simulink model "robot_model_with_torque"  (R2018b)
settings: Solver=VariableStepAuto  StartTime=0.0  StopTime=25  RelTol=1e-6
model workspace: external: MATLAB File load_data.m (data not in the file)
values from neighbouring files (symbols this model uses):
  m = [5.70044 3.22698 4.31272 2.07206 2.24665 1.60879]    [init_robot.m]    (also in load_data.m)
  smiData = struct    [load_data.m]
undefined symbols (not defined in the file or in its folder): X, Y, Z
libraries: sm_lib x40, nesl_utility x15, simulink x1
(part 2 of 2)

== matlab function robot_model_with_torque/motores1/MATLAB Function5 ==
  data: E output; Y input; dY input; iE input; U output; Yref input; dYref input; k input
function [E,U] = PID(Y,dY,iE,Yref,dYref,k)

E = Yref - Y;
dE = dYref - dY;

U = k(1)*E + k(2)*iE + k(3)*dE;

== matlab function robot_model_with_torque/motores1/MATLAB Function6 ==
  data: U input; D input; dX output; Y output; X input
function [dX,Y]= motor_modelo(U,D,X)

%MATRICES DEL MOTOR
Ra = 11.24;
La = 2.713e-3;
Kb = 14.87e-3;
Kt = Kb;
bm = 2.01e-6;
Jm = 2779.56e-9;

A = [-Ra/La -Kb/La;Kt/Jm -bm/Jm];
B = [1/La;0];
C = [0 1];

%CONTROLADOR PID
dX = [A*X + B*U];
Y = [C*X + D*U];

== matlab function robot_model_with_torque/motores1/MATLAB Function7 ==
  data: E output; Y input; dY input; iE input; U output; Yref input; dYref input; k input
function [E,U] = PID(Y,dY,iE,Yref,dYref,k)

E = Yref - Y;
dE = dYref - dY;

U = k(1)*E + k(2)*iE + k(3)*dE;

== matlab function robot_model_with_torque/motores1/MATLAB Function8 ==
  data: U input; D input; dX output; Y output; X input
function [dX,Y]= motor_modelo(U,D,X)

%MATRICES DEL MOTOR
Ra = 11.24;
La = 2.713e-3;
Kb = 14.87e-3;
Kt = Kb;
bm = 2.01e-6;
Jm = 2779.56e-9;

A = [-Ra/La -Kb/La;Kt/Jm -bm/Jm];
B = [1/La;0];
C = [0 1];

%CONTROLADOR PID
dX = [A*X + B*U];
Y = [C*X + D*U];

== matlab function robot_model_with_torque/motores1/MATLAB Function9 ==
  data: w output; q input; dq input; torque output; ddq input; dw input
function [w,torque] = fcn(q, dq, ddq, dw)

d = [0.2703 0 0.3644 0 0.3743 0 0.2295]; %metros
a = [0.069 0 0.069 0 0.01 0 0]; %matros
alpha = [-pi/2 pi/2 -pi/2 pi/2 -pi/2 pi/2 0]; %radianes
m = [5.70044 3.22698 4.31272 2.07206 2.24665 1.60879 0.54218]; %kg

xc = [-0.05117 0.00269 -0.07176 0.00159 -0.01168 0.00697 0.005137]; %metros
yc = [0.07908 -0.00529 0.08149 -0.01117 0.13111 0.006 0.0009572];
zc = [0.00086 0.06845 0.00132 0.02618 0.0046 0.06048 0.0-6682];

%Tensores de inercia (kg*m^2)
Ixx = [0.047091023 0.027885975 0.026617336 0.013182279 0.016677428 0.007005379 0.000816214];
Iyy = [0.035959884 0.020787492 0.012480083 0.00926852 0.003746311 0.005527552 0.000873501];
Izz = [0.037669765 0.011752094 0.028443552 0.007115827 0.016754573 0.003876072 0.000549415];
Ixy = [-0.0061487 -0.00018822 -0.003921899 -0.000196634 -0.000186576 0.000153481 0.00012844];
Iyx = [-0.0061487 -0.00018822 -0.003921899 -0.000196634 -0.000186576 0.000153481 0.00012844];
Iyz = [-0.000780869 0.002076758 -0.001083893 0.000745949 0.000647324 -0.00021115 0.000105773];
Izy = [-0.000780869 0.002076758 -0.001083893 0.000745949 0.000647324 -0.00021115 0.000105773];
Ixz = [0.000127876 -0.000300964 0.000292706 0.000360362 0.000184037 -0.000443848 0.000189699];
Izx = [0.000127876 -0.000300964 0.000292706 0.000360362 0.000184037 -0.000443848 0.000189699];

Ti = denavit_hartenberg(q,a,alpha,d,0,7);
rici = zeros(3,7);
rmci = zeros(3,7);
rimi = zeros(3,7);

for i = 1:7
    rici(:,i) = Ti{i}(1:3,4)- [xc(i);yc(i);zc(i)];
end

for i = 1:6
    rmci(:,i) = Ti{i + 1}(1:3,4)- Ti{i}(1:3,4) - [xc(i);yc(i);zc(i)];
end

for i = 1:6
    rimi(:,i) = Ti{i + 1}(1:3,4) - Ti{i}(1:3,4);
end

T0 = denavit_hartenberg(q,a,alpha,d,0,7);

w = zeros(3,7);
aw = zeros(3,7);
ac = zeros(3,7);
ae = zeros(3,7);
f = zeros(3,7);
g = zeros(3,7);
Tq = zeros(3,7);
torque = zeros(7,1);

%w1
Ri = Ti{1}(1:3,1:3);
Z0 = [0;0;1];
bi = Ri'*Z0;
w(:,1) = bi*dq(1);
aw(:,1) = bi*ddq(1) + cross(w(:,1),bi*dq(1));
ae(:,1) = cross(dw(:,1),rimi(:,1)) + cross(w(:,1),cross(w(:,1),rimi(:,1)));
ac(:,1) = cross(dw(:,1),rici(:,1)) + cross(w(:,1),cross(w(:,1),rici(:,1)));
g(:,1) = -Ri'*9.78*[0;0;1];

for i = 2:7
   Ri = Ti{i}(1:3,1:3); 
   Rmi = [dot(Ti{i}(1,4),Ti{i-1}(1,4)) dot(Ti{i}(2,4),Ti{i-1}(1,4)) dot(Ti{i}(3,4),Ti{i-1}(1,4));...
       dot(Ti{i}(1,4),Ti{i-1}(2,4)) dot(Ti{i}(2,4),Ti{i-1}(2,4)) dot(Ti{i}(3,4),Ti{i-1}(2,4));...
       dot(Ti{i}(1,4),Ti{i-1}(3,4)) dot(Ti{i}(2,4),Ti{i-1}(3,4)) dot(Ti{i}(3,4),Ti{i-1}(3,4))]';
   bi = Ri'*Ti{i - 1}(1:3,3);
   w(:,i) = Rmi'*w(:,i-1) + bi*dq(i);
   aw(:,i) = Rmi'*aw(:,i-1) +bi*ddq(i) + cross(w(:,i),bi*dq(i));
   ae(:,i) = Rmi'*ae(:,i-1) + cross(dw(:,i),rimi(:,i)) + cross(w(:,i),cross(w(:,i),rimi(:,i)));
   ac(:,i) = Rmi'*ac(:,i-1) + cross(dw(:,i),rici(:,i)) + cross(w(:,i),cross(w(:,i),rici(:,i)));
   g(:,i) = -Ri'*9.78*[0;0;1];
end

%f7
f(:,7) = m(7)*ac(:,7) - m(7)*g(:,7);
I = [Ixx(7) Ixy(7) Ixz(7);Iyx(7) Iyy(7) Iyz(7);Izx(7) Izy(7) Izz(7)];
Tq(:,7) = - cross(f(:,7),rici(:,7)) + aw(:,7) + cross(w(:,7),I*w(:,7));
torque(7) = sqrt(Tq(1,7)^2 + Tq(2,7)^2 + Tq(3,7)^2);

for i = 6:-1:1
    Rmi = [dot(Ti{i + 1}(1,4),Ti{i}(1,4)) dot(Ti{i + 1}(2,4),Ti{i}(1,4)) dot(Ti{i+1}(3,4),Ti{i}(1,4));...
       dot(Ti{i+1}(1,4),Ti{i}(2,4)) dot(Ti{i+1}(2,4),Ti{i}(2,4)) dot(Ti{i+1}(3,4),Ti{i}(2,4));...
       dot(Ti{i+1}(1,4),Ti{i}(3,4)) dot(Ti{i+1}(2,4),Ti{i}(3,4)) dot(Ti{i+1}(3,4),Ti{i}(3,4))]';
   I = [Ixx(i) Ixy(i) Ixz(i);Iyx(i) Iyy(i) Iyz(i);Izx(i) Izy(i) Izz(i)];
   f(:,i) = Rmi*f(:,i+1) + m(i)*ac(:,i) - m(i)*g(:,i);
   Tq(:,i) = Rmi*Tq(:,i+1) - cross(f(:,i),rici(:,i)) + cross(Rmi*f(:,i+1),rmci(:,i)) + aw(:,i) + cross(w(:,i),I*w(:,i));
   torque(i) = sqrt(Tq(1,i)^2 + Tq(2,i)^2 + Tq(3,i)^2);
end
